simulink model "EletroIma_com_Solenoide"  (R2018b)
settings: Solver=VariableStepAuto  StartTime=0.0  StopTime=12  RelTol=1e-3
model workspace (MAT data in the model file):
  Var = 0
settings Model: Creator=Leonardo LASID  LastModifiedBy=Leonardo LASID

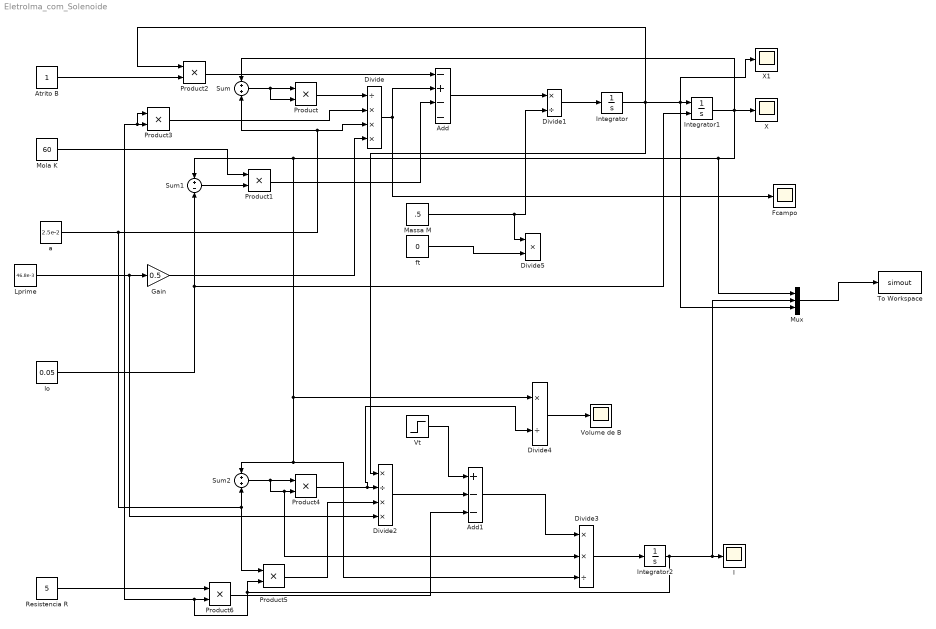
== system EletroIma_com_Solenoide ==
  Add : Sum  Inputs=-+--
  Add1 : Sum  Inputs=+--
  Atrito B : Constant
  Divide : Product  Inputs=/***
  Divide1 : Product  Inputs=*/
  Divide2 : Product  Inputs=*/**
  Divide3 : Product  Inputs=**/
  Divide4 : Product  Inputs=*/
  Divide5 : Product  Inputs=**
  "Fcampo " : Scope
  Gain : Gain  Gain=0.5
  I : Scope
  Integrator : Integrator
  Integrator1 : Integrator  InitialConditionSource=external
  Integrator2 : Integrator
  Lprime : Constant  Value=46.8e-3
  Massa M : Constant  Value=.5
  Mola K : Constant  Value=60
  Mux : Mux  Inputs=3
  Product{,1..6} (7 alike) : Product
  Resistencia R : Constant  Value=5
  Sum : Sum
  Sum1 : Sum  Inputs=+-
  Sum2 : Sum
  To Workspace : ToWorkspace  VariableName=simout  SaveFormat=Timeseries  SampleTime=-1
  Volume de B : Scope
  Vt : Step  Time=0.5  After=10  SampleTime=0
  X : Scope
  X1 : Scope
  a : Constant  Value=2.5e-2
  ft : Constant  Value=0
  lo : Constant  Value=0.05
  wires:
  Add/1 -> Divide1/1
  Divide/1 -> Add/2, "Fcampo "/1
  Product/1 -> Divide/1
  Sum/1 -> Product/2, Product/1
  Product1/1 -> Add/3
  Sum1/1 -> Product1/2
  Product2/1 -> Add/1
  Product3/1 -> Divide/2
  Gain/1 -> Divide/4
  Divide1/1 -> Integrator/1
  Integrator/1 -> Divide2/1, Mux/3, X1/1, Integrator1/1, Product2/1
  Integrator1/1 -> Sum/1, Mux/1, Sum1/1, Divide4/1, Divide3/3, Sum2/1, X/1
  Atrito B/1 -> Product2/2
  Mola K/1 -> Product1/1
  lo/1 -> Sum1/2, Integrator1/2
  Massa M/1 -> Divide5/1, Divide1/2
  Lprime/1 -> Gain/1, Divide2/4
  a/1 -> Divide/3, Sum/2, Product5/1, Sum2/2
  Divide2/1 -> Add1/2
  Add1/1 -> Divide3/1
  Divide3/1 -> Integrator2/1
  Integrator2/1 -> Product3/1, Product3/2, Product6/2, Product5/2, Mux/2, I/1
  Sum2/1 -> Divide3/2, Product4/2, Product4/1
  Product4/1 -> Divide4/2, Divide2/2
  Product5/1 -> Divide2/3
  Resistencia R/1 -> Product6/1
  Product6/1 -> Add1/3
  Vt/1 -> Add1/1
  Mux/1 -> To Workspace/1
  Divide4/1 -> Volume de B/1
  ft/1 -> Divide5/2
